simulink model "AC_base_1_VSM_2"  (R2023a)
settings: Solver=ode3  StartTime=0.0  StopTime=8  FixedStep=HWSampleTime  RelTol=1e-3
values from neighbouring files (symbols this model uses):
  ControlSampleTime = 1/8000    (= 0.000125)    [initTPHardware.m]
  HWSampleTime = ControlSampleTime / Oversample    [Sim_TP3_VSM_init.m]    (also in initTPHardware.m = 3.125e-05)
  Ipwm_back = 1.2    [Sim_TP3_VSM_init.m]
  Ipwm_off = 1.2    [Sim_TP3_VSM_init.m]
  Oversample = 1    [Sim_TP3_VSM_init.m]
  scaling_factor = 1/15e4    (= 6.66666666667e-06)    [Sim_TP3_VSM_init.m]
  SM = initStateMachine(EXEC_MODE)    [Sim_TP3_VSM_init.m]
  Ts = ControlSampleTime    [Sim_TP3_VSM_init.m]
  V_DC = 720    [Sim_TP3_VSM_init.m]
undefined symbols (not defined in the file or in its folder): DiscIntNeverNeededParam, LCL, Manage, Param, VSMCTRL
libraries: fl_lib x100, nesl_utility x63, simulink x38, FriedrichLibrary x38, ee_lib x20, simulink_extras x14, TriphaseHardwaremodule x12, spsEdgeDetectorLib x2, StateMachines x2, slpidlib x2, spsPower3phInstantaneousLib x1
(part 3 of 7)

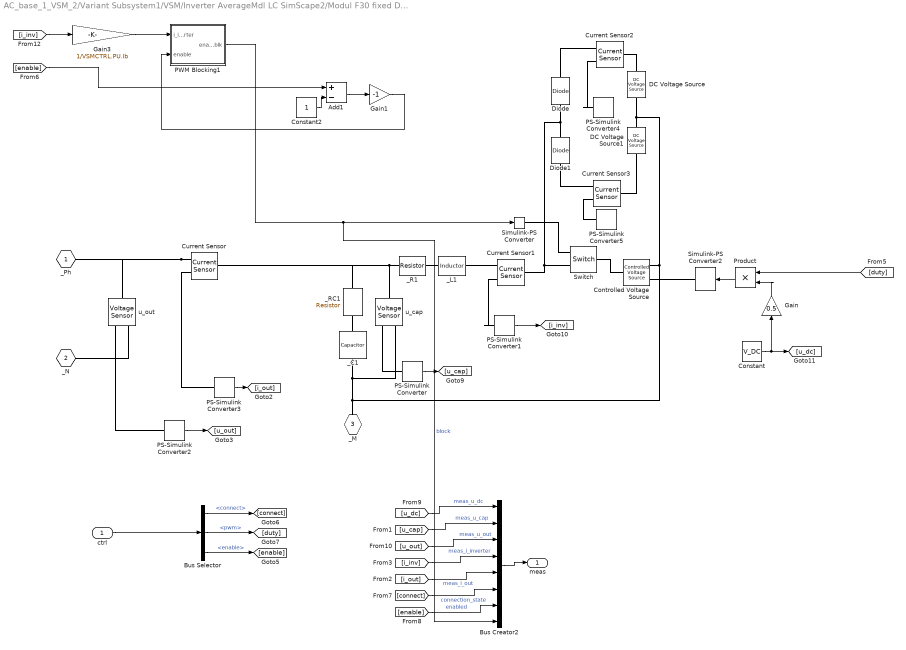
== system AC_base_1_VSM_2/Variant Subsystem1/VSM/Inverter AverageMdl LC SimScape2/Modul F30 fixed DC voltage Average SimScape/simscape_bridgefilter_aca2 ==
  ctrl : Inport
  Add1 : Sum  Inputs=+-
  Bus Creator2 : BusCreator  Inputs=8
  Bus Selector : BusSelector  OutputSignals=connect,pwm,enable
  Constant : Constant  Value=V_DC
  Constant2 : Constant
  Controlled Voltage Source : fl_lib/Electrical/Electrical Sources/Controlled Voltage Source
  Current Sensor{,1..3} (4 alike) : fl_lib/Electrical/Electrical Sensors/Current Sensor
  DC Voltage Source : fl_lib/Electrical/Electrical Sources/DC Voltage Source  v0=V_DC/2 V
  DC Voltage Source1 : fl_lib/Electrical/Electrical Sources/DC Voltage Source  v0=V_DC/2 V
  Diode : fl_lib/Electrical/Electrical Elements/Diode  Vf=0.6 V  Ron=0.001*scaling_factor Ohm  Goff=1e-8 1/Ohm  i_specify=off  i_priority=None  i=0 A  i_nominal_specify=off  i_nominal_unit=A  i_nominal_value=1  v_specify=off  v_priority=None  v=0 V  v_nominal_specify=off  v_nominal_unit=V  v_nominal_value=1
  Diode1 : fl_lib/Electrical/Electrical Elements/Diode  Vf=0.6 V  Ron=0.001*scaling_factor Ohm  Goff=1e-8 1/Ohm  i_specify=off  i_priority=None  i=0 A  i_nominal_specify=off  i_nominal_unit=A  i_nominal_value=1  v_specify=off  v_priority=None  v=0 V  v_nominal_specify=off  v_nominal_unit=V  v_nominal_value=1
  Gain : Gain  Gain=0.5
  Gain1 : Gain  Gain=-1
  Gain3 : Gain  Gain=1/VSMCTRL.PU.Ib
  PS-Simulink Converter{,1..5} (6 alike) : nesl_utility/PS-Simulink Converter  PhysicalDomain=network_engine_domain  SubClassName=ps_output  LeftPortType=input  RightPortType=output  PseudoPeriodic=off  Frequencies=[]  VectorFormat=1-D array  Unit=1  AffineConversion=off
  PWM Blocking1 : Subsystem
  Product : Product
  Simulink-PS Converter : nesl_utility/Simulink-PS Converter  PhysicalDomain=network_engine_domain  SubClassName=ps_input  LeftPortType=input  RightPortType=output  PseudoPeriodic=off  Frequencies=[]  NoiseDistribution=none  NoiseParameters=[]  Unit=1  AffineConversion=off  FilteringAndDerivatives=provide  SimscapeFilterOrder=1  InputFilterTimeConstant=0.001  UdotUserProvided=0
  Simulink-PS Converter2 : nesl_utility/Simulink-PS Converter  PhysicalDomain=network_engine_domain  SubClassName=ps_input  LeftPortType=input  RightPortType=output  PseudoPeriodic=off  Frequencies=[]  NoiseDistribution=none  NoiseParameters=[]  Unit=1  AffineConversion=off  FilteringAndDerivatives=zero  SimscapeFilterOrder=1  InputFilterTimeConstant=0.001  UdotUserProvided=1
  Switch : fl_lib/Electrical/Electrical Elements/Switch  R_closed=0.001*scaling_factor Ohm  G_open=1e-8 1/Ohm  Threshold=0.5  i_specify=off  i_priority=None  i=0 A  i_nominal_specify=off  i_nominal_unit=A  i_nominal_value=1  v_specify=off  v_priority=None  v=0 V  v_nominal_specify=off  v_nominal_unit=V  v_nominal_value=1
  _C1 : fl_lib/Electrical/Electrical Elements/Capacitor  c=C1 F  r=1e-6 Ohm  g=0 1/Ohm  i_specify=off  i_priority=None  i=0 A  i_nominal_specify=off  i_nominal_unit=A  i_nominal_value=1  v_specify=off  v_priority=None  v=0 V  v_nominal_specify=off  v_nominal_unit=V  v_nominal_value=1  vc_specify=off  vc_priority=None  vc=0 V  vc_nominal_specify=off  vc_nominal_unit=V  vc_nominal_value=1
  _L1 : fl_lib/Electrical/Electrical Elements/Inductor  l=L1 H  r=0 Ohm  g=1e-9 1/Ohm  i_specify=off  i_priority=None  i=0 A  i_nominal_specify=off  i_nominal_unit=A  i_nominal_value=1  v_specify=off  v_priority=None  v=0 V  v_nominal_specify=off  v_nominal_unit=V  v_nominal_value=1  i_L_specify=off  i_L_priority=None  i_L=0 A  i_L_nominal_specify=off  i_L_nominal_unit=A  i_L_nominal_value=1
  _R1 : fl_lib/Electrical/Electrical Elements/Resistor  R=R_L1 Ohm  i_specify=off  i_priority=None  i=0 A  i_nominal_specify=off  i_nominal_unit=A  i_nominal_value=1  v_specify=off  v_priority=None  v=0 V  v_nominal_specify=off  v_nominal_unit=V  v_nominal_value=1
  _RC1 : fl_lib/Electrical/Electrical Elements/Resistor  R=R_C1 Ohm  i_specify=off  i_priority=None  i=0 A  i_nominal_specify=off  i_nominal_unit=A  i_nominal_value=1  v_specify=off  v_priority=None  v=0 V  v_nominal_specify=off  v_nominal_unit=V  v_nominal_value=1
  u_cap : fl_lib/Electrical/Electrical Sensors/Voltage Sensor
  u_out : fl_lib/Electrical/Electrical Sensors/Voltage Sensor
  _Ph : PMIOPort  Side=Left
  _N : PMIOPort  Port=2  Side=Left
  _M : PMIOPort  Port=3  Side=Right
  meas : Outport  VectorParamsAs1DForOutWhenUnconnected=off
  wires:
  Gain1/1 -> PWM Blocking1/2(enable)
  [enable] -> Add1/1
  PWM Blocking1/1(enable_blk) -> Simulink-PS Converter/1, Bus Creator2/8  "block"
  [i_inv] -> Gain3/1
  Gain3/1 -> PWM Blocking1/1(i_inverter)
  Add1/1 -> Gain1/1
  Constant2/1 -> Add1/2
  PS-Simulink Converter3/1 -> [i_out]
  Gain/1 -> Product/2
  [duty] -> Product/1
  Constant/1 -> Gain/1, [u_dc]
  Product/1 -> Simulink-PS Converter2/1
  PS-Simulink Converter2/1 -> [u_out]
  PS-Simulink Converter1/1 -> [i_inv]
  PS-Simulink Converter/1 -> [u_cap]
  [u_dc] -> Bus Creator2/1  "meas_u_dc"
  Bus Creator2/1 -> meas/1
  [enable] -> Bus Creator2/7  "enabled"
  Bus Selector/3 -> [enable]  "<enable>"
  [u_cap] -> Bus Creator2/2  "meas_u_cap"
  [u_out] -> Bus Creator2/3  "meas_u_out"
  [i_inv] -> Bus Creator2/4  "meas_i_inverter"
  [i_out] -> Bus Creator2/5  "meas_i_out"
  ctrl/1 -> Bus Selector/1
  [connect] -> Bus Creator2/6  "connection_state"
  Bus Selector/1 -> [connect]  "<connect>"
  Bus Selector/2 -> [duty]  "<pwm>"
  connections:
  Current Sensor2/LConn1 -- DC Voltage Source/LConn1
  PS-Simulink Converter5/LConn1 -- Current Sensor3/RConn1
  Current Sensor2/RConn2 -- Diode/RConn1
  PS-Simulink Converter4/LConn1 -- Current Sensor2/RConn1
  Current Sensor3/RConn2 -- Diode1/LConn1
  Current Sensor3/LConn1 -- DC Voltage Source1/RConn1
  Simulink-PS Converter/RConn1 -- Switch/RConn1
  Controlled Voltage Source/LConn1 -- Switch/LConn1
  Diode/LConn1 -- Switch/RConn2 -- Current Sensor1/LConn1 -- Diode1/RConn1
  _RC1/RConn1 -- _C1/LConn1
  PS-Simulink Converter3/LConn1 -- Current Sensor/RConn1
  PS-Simulink Converter2/LConn1 -- u_out/RConn1
  PS-Simulink Converter1/LConn1 -- Current Sensor1/RConn1
  PS-Simulink Converter/LConn1 -- u_cap/RConn1
  Simulink-PS Converter2/RConn1 -- Controlled Voltage Source/RConn1
  u_out/RConn2 -- _N/RConn1
  Current Sensor/RConn2 -- _Ph/RConn1 -- u_out/LConn1
  DC Voltage Source1/LConn1 -- Controlled Voltage Source/RConn2 -- _C1/RConn1 -- u_cap/RConn2 -- _M/RConn1 -- DC Voltage Source/RConn1
  _R1/LConn1 -- u_cap/LConn1 -- Current Sensor/LConn1 -- _RC1/LConn1
  Current Sensor1/RConn2 -- _L1/RConn1
  _R1/RConn1 -- _L1/LConn1

== system AC_base_1_VSM_2/Variant Subsystem1/VSM/VSM1/VSM/BUS_GENERATION ==
  MANAGE : Inport
  CONTROL : Inport  Port=2
  Bus Creator1 : BusCreator  Inputs=4
  Bus Selector2 : BusSelector  OutputSignals=PWM
  Bus Selector3 : BusSelector  OutputSignals=ENABLED,CONNECT
  Bus Selector4 : BusSelector  OutputSignals=CONNECTED,ENABLED
  Bus Creator6 : BusCreator  Inputs=2  OutDataTypeStr=Bus: FeedbackACBus
  Data Type Conversion{,1..3} (4 alike) : DataTypeConversion  SaturateOnIntegerOverflow=off  RndMeth=Floor
  Signal Specification1 : SignalSpecification
  additional data1 : Constant  Value=0
  ctrl : Outport  VectorParamsAs1DForOutWhenUnconnected=off
  feedback : Outport  Port=2  VectorParamsAs1DForOutWhenUnconnected=off
  wires:
  Bus Selector2/1 -> Signal Specification1/1  "<PWM>"
  Bus Selector4/1 -> Data Type Conversion3/1  "<CONNECTED>"
  Bus Selector4/2 -> Data Type Conversion2/1  "<ENABLED>"
  CONTROL/1 -> Bus Selector2/1
  Data Type Conversion2/1 -> Bus Creator6/2  "enabled"
  Signal Specification1/1 -> Bus Creator1/1  "pwm"
  MANAGE/1 -> Bus Selector3/1, Bus Selector4/1
  Bus Creator1/1 -> ctrl/1
  Bus Creator6/1 -> feedback/1
  Bus Selector3/1 -> Data Type Conversion/1  "<ENABLED>"
  Data Type Conversion/1 -> Bus Creator1/2  "enable"
  Data Type Conversion1/1 -> Bus Creator1/3  "connect"
  additional data1/1 -> Bus Creator1/4  "source_id"
  Bus Selector3/2 -> Data Type Conversion1/1  "<CONNECT>"
  Data Type Conversion3/1 -> Bus Creator6/1  "connected"

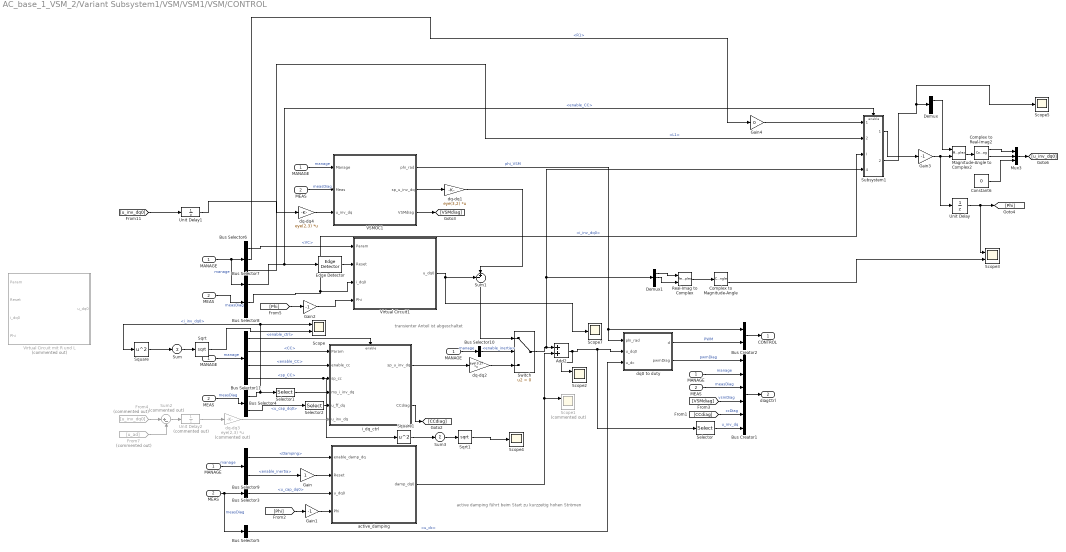
== system AC_base_1_VSM_2/Variant Subsystem1/VSM/VSM1/VSM/CONTROL ==
  note: transienter Anteil ist abgeschaltet
  note: active damping führt beim Start zu kurzzeitig hohen Strömen
  MANAGE : Inport
  MEAS : Inport  Port=2
  "  MANAGE " : InportShadow
  "  MEAS " : InportShadow  Port=2
  "  MEAS  " : InportShadow  Port=2
  " MANAGE" : InportShadow
  " MEAS" : InportShadow  Port=2
  Add2 : Sum
  Bus Creator1 : BusCreator  Inputs=6
  Bus Creator2 : BusCreator  Inputs=2
  Bus Selector10 : BusSelector  OutputSignals=enable_VSM.enable_inertia
  Bus Selector11 : BusSelector  OutputSignals=enable_VSM.enable_ctrl,Param.CC,enable_CC,sp_CC
  Bus Selector3 : BusSelector  OutputSignals=u_cap.u_cap_dq0
  Bus Selector4 : BusSelector  OutputSignals=i_inv.i_inv_dq0,u_cap.u_cap_dq0
  Bus Selector5 : BusSelector  OutputSignals=u_dc
  Bus Selector6 : BusSelector  OutputSignals=Param.VC,Param.VC.R1,Param.VC.L1
  Bus Selector7 : BusSelector  OutputSignals=enable_CC
  Bus Selector8 : BusSelector  OutputSignals=i_inv.i_inv_dq0
  Bus Selector9 : BusSelector  OutputSignals=Param.Damping,enable_VSM.enable_inertia
  Complex to Magnitude-Angle : ComplexToMagnitudeAngle
  Complex to Real-Imag2 : ComplexToRealImag
  Constant6 : Constant  Value=0
  Demux : Demux  Outputs=2
  Demux1 : Demux  Outputs=3
  Edge Detector : spsEdgeDetectorLib/Edge Detector  model=Falling  ic=0  Ts=0
  From4 : From  Commented=on  GotoTag=u_inv_dq0
  From7 : From  Commented=on  GotoTag=u_ad
  Gain : Gain
  Gain1 : Gain  Gain=-1
  Gain2 : Gain  Gain=-1
  Gain3 : Gain  Gain=-1
  Gain4 : Gain  Gain=0
  "MANAGE  " : InportShadow
  "MANAGE   " : InportShadow
  "MANAGE    " : InportShadow
  "MEAS " : InportShadow  Port=2
  Magnitude-Angle to Complex2 : MagnitudeAngleToComplex
  Mux3 : Mux  Inputs=3
  Real-Imag to Complex : RealImagToComplex
  Scope : Scope  NumInputPorts=2
  Scope1 : Scope  Commented=on  NumInputPorts=2
  Scope2 : Scope  NumInputPorts=2
  Scope3 : Scope  NumInputPorts=2
  Scope4 : Scope
  Scope5 : Scope
  Scope7 : Scope  NumInputPorts=3
  Selector : Selector  InputPortWidth=3  IndexOptions=Index vector (dialog)  Indices=[1 2]  OutputSizes=1
  Selector1 : Selector  InputPortWidth=3  IndexOptions=Index vector (dialog)  Indices=[1 2]  OutputSizes=1
  Selector2 : Selector  InputPortWidth=3  IndexOptions=Index vector (dialog)  Indices=[1 2]  OutputSizes=1
  Sqrt : Sqrt
  Sqrt1 : Sqrt
  Square : Math  Operator=square
  Square1 : Math  Operator=square
  Subsystem1 : Subsystem
  Sum : Sum  Inputs=+
  Sum1 : Sum  Inputs=-+|
  Sum2 : Sum  Commented=on  Inputs=|+-
  Sum3 : Sum  Inputs=+
  Switch : Switch  Criteria=u2 > Threshold  SaturateOnIntegerOverflow=off  InputSameDT=off
  Unit Delay : UnitDelay  SampleTime=-1  HasFrameUpgradeWarning=on
  Unit Delay1 : UnitDelay  SampleTime=ControlSampleTime  HasFrameUpgradeWarning=on
  Unit Delay2 : UnitDelay  Commented=on  SampleTime=ControlSampleTime  HasFrameUpgradeWarning=on
  VSMOC1 : Subsystem  mask(VSM mit OC){VSM=Ctrl.VSM}
      mask prompts: VSM "VSM Parameter"
      mask help:
      | VSM(.Ta, .kpf, .kdf, .f0, .ku, .Tu)
      |
      | Parameter nicht auf der Maske:
      | ControlSampleTime
  Virtual Circuit mit R und L : Subsystem  Commented=on  AncestorBlock=ControLibrary/Virtual Circuit
      settings: LibrarySourceBlock=ControLibrary/Virtual Circuit
  Virtual Circuit1 : Subsystem  AncestorBlock=ControLibrary/Virtual Circuit
      settings: LibrarySourceBlock=ControLibrary/Virtual Circuit
  active_damping : Subsystem  mask(Lead Lag){OmLead=Ctrl.VTFF.OmLead, OmLag=Ctrl.VTFF.OmLag}
      mask prompts: OmLead "Omega Lead"; OmLag "Omega Lag"
  dq-dq1 : Gain  Gain=eye(3,2)  Multiplication=Matrix(K*u)
  dq-dq2 : Gain  Gain=eye(3,2)  Multiplication=Matrix(K*u)
  dq-dq3 : Gain  Commented=on  Gain=eye(2,3)  Multiplication=Matrix(K*u)
  dq-dq4 : Gain  Gain=eye(2,3)  Multiplication=Matrix(K*u)
  dq0 to duty : Subsystem
  i_dq_ctrl : Subsystem  mask(PI DQ Stromregler){Kp=Ctrl.CC.kp*0+0.28*2.5/2, Ki=Ctrl.CC.ki*0+28*20/2, L_inv=Ctrl.CC.xff, Kff=Ctrl.CC.Kff}
      mask prompts: Kp "P-Anteil:"; Ki "I-Anteil:"; L_inv "Induktivität [pu]:"; Kff "Vorsteuerung"
      mask help:
      | - in pu Einheiten
      | - 2-phasige DQ Regelung
      | - Entkopplung der d- und q-Achse
      | - Vorsteuerung der Kondensatorspannung
      | - Aktive Dämpfung der LC-Filter Resonanz
      | - Aktive Dämpfung der Zwischenkreis Spannung
  CONTROL : Outport  VectorParamsAs1DForOutWhenUnconnected=off
  diagCtrl : Outport  Port=2  VectorParamsAs1DForOutWhenUnconnected=off
  wires:
  Square1/1 -> Sum3/1
  Sum3/1 -> Sqrt1/1
  Sqrt1/1 -> Scope4/1
  Complex to Magnitude-Angle/2 -> Scope3/2
  Real-Imag to Complex/1 -> Complex to Magnitude-Angle/1
  Demux1/1 -> Real-Imag to Complex/1
  Demux1/2 -> Real-Imag to Complex/2
  Unit Delay/1 -> [Phi], Scope3/1
  Sqrt/1 -> Scope/2
  Sum/1 -> Sqrt/1
  Square/1 -> Sum/1
  Gain4/1 -> Subsystem1/1(<R1>)
  Edge Detector/1 -> Virtual Circuit1/2(Reset)
  Demux/1 -> Magnitude-Angle to Complex2/1
  active_damping/1(damp_dq0) -> Add2/2, Scope1/1
  Complex to Real-Imag2/2 -> Mux3/2
  Complex to Real-Imag2/1 -> Mux3/1
  Switch/1 -> Add2/1, Subsystem1/4(U_i), Demux1/1
  i_dq_ctrl/1(sp_u_inv_dq) -> dq-dq2/1
  Gain3/1 -> Magnitude-Angle to Complex2/2, Unit Delay/1
  dq-dq4/1 -> VSMOC1/3(u_inv_dq)
  Subsystem1/2(U_v) -> Demux/1, Scope5/1
  Subsystem1/1(phi_vsm) -> Gain3/1
  dq-dq1/1 -> Sum1/2
  Mux3/1 -> [u_inv_dq0]
  Constant6/1 -> Mux3/3
  Magnitude-Angle to Complex2/1 -> Complex to Real-Imag2/1
  [u_inv_dq0] -> Unit Delay1/1
  Bus Selector6/3 -> Subsystem1/2(<L1>)  "<L1>"
  Bus Selector6/2 -> Gain4/1  "<R1>"
  Virtual Circuit1/1(" u_dq0") -> Sum1/1, Scope7/2
  Bus Selector7/1 -> Subsystem1/Enable, Edge Detector/1  "<enable_CC>"
  Bus Selector8/1 -> Subsystem1/3(I), Virtual Circuit1/3(i_dq0)  "<i_inv_dq0>"
  Bus Selector11/4 -> i_dq_ctrl/3(sp_cc), Square1/1  "<sp_CC>"
  Selector1/1 -> i_dq_ctrl/4(ms_i_inv_dq)
  Bus Selector4/2 -> Selector2/1  "<u_cap_dq0>"
  Bus Selector11/3 -> i_dq_ctrl/2(enable_cc)  "<enable_CC>"
  Gain2/1 -> Virtual Circuit1/4(Phi)
  [Phi] -> Gain2/1
  From7/1 -> Sum2/2
  From4/1 -> Sum2/1
  Sum2/1 -> Unit Delay2/1
  Gain1/1 -> active_damping/4(Phi)
  Gain/1 -> active_damping/2(Reset)
  Bus Selector9/2 -> Gain/1  "<enable_inertia>"
  Bus Selector3/1 -> active_damping/3(u_dq0)  "<u_cap_dq0>"
  Unit Delay2/1 -> dq-dq3/1
  VSMOC1/1(phi_rad) -> dq0 to duty/1(phi_rad), Bus Creator2/1  "phi_VSM"
  Bus Selector6/1 -> Virtual Circuit1/1(Param)  "<VC>"
  "MANAGE   "/1 -> Bus Selector6/1, Bus Selector7/1  "manage"
  "  MEAS  "/1 -> Bus Selector8/1  "measDiag"
  Selector/1 -> Bus Creator1/6  "u_inv_dq"
  VSMOC1/2(sp_u_inv_dq) -> dq-dq1/1
  Bus Selector5/1 -> dq0 to duty/3(u_dc)  "<u_dc>"
  [CCdiag] -> Bus Creator1/5  "ccDiag"
  "MANAGE  "/1 -> Bus Selector10/1  "manage"
  Bus Selector10/1 -> Switch/2  "<enable_inertia>"
  i_dq_ctrl/2(CCdiag) -> [CCdiag]
  Bus Selector4/1 -> Selector1/1, Scope/1, Square/1  "<i_inv_dq0>"
  "MEAS "/1 -> Bus Selector4/1  "measDiag"
  "MANAGE    "/1 -> Bus Selector11/1  "manage"
  Bus Selector11/1 -> i_dq_ctrl/Enable  "<enable_ctrl>"
  Selector2/1 -> i_dq_ctrl/5(u_ff_dq)
  Bus Selector11/2 -> i_dq_ctrl/1(Param)  "<CC>"
  dq-dq3/1 -> i_dq_ctrl/6(u_inv_dq)
  Add2/1 -> dq0 to duty/2(u_dq0), Selector/1, Scope2/1
  MEAS/1 -> VSMOC1/2(Meas)  "measDiag"
  Bus Creator2/1 -> CONTROL/1
  " MEAS"/1 -> Bus Selector5/1, Bus Selector3/1  "measDiag"
  "  MANAGE "/1 -> Bus Creator1/2  "manage"
  Bus Creator1/1 -> diagCtrl/1
  Bus Selector9/1 -> active_damping/1(enable_damp_dq)  "<Damping>"
  " MANAGE"/1 -> Bus Selector9/1  "manage"
  dq0 to duty/2(pwmDiag) -> Bus Creator1/1  "pwmDiag"
  MANAGE/1 -> VSMOC1/1(Manage)  "manage"
  dq0 to duty/1(d) -> Bus Creator2/2  "PWM"
  VSMOC1/3(VSMdiag) -> [VSMdiag]
  "  MEAS "/1 -> Bus Creator1/3  "measDiag"
  [VSMdiag] -> Bus Creator1/4  "vsmDiag"
  Sum1/1 -> Switch/1
  dq-dq2/1 -> Switch/3
  Unit Delay1/1 -> dq-dq4/1
  [Phi] -> Gain1/1

== system AC_base_1_VSM_2/Variant Subsystem1/VSM/VSM1/VSM/MANAGEMENT ==
  CMD : Inport
  MEAS : Inport  Port=2
  "    MEAS   " : InportShadow  Port=2
  "  CMD  " : InportShadow
  " CMD" : InportShadow
  Add : Sum
  Bus Creator4 : BusCreator  Inputs=8
  Bus Creator5 : BusCreator  Inputs=2
  Bus Selector1 : BusSelector  OutputSignals=Param
  Bus Selector3 : BusSelector  OutputSignals=i_inv.i_inv_ab0,i_inv.i_inv_dq0
  Bus Selector7 : BusSelector  OutputSignals=i_inv.i_inv_dq0,PQ,u_cap.u_cap_ab0,PQ_out,i_out.i_out_ab0
  Bus Selector10 : BusSelector  OutputSignals=Param.CC.i_sp_gain
  Bus Selector11 : BusSelector  OutputSignals=Manage.enable
  Bus Selector12 : BusSelector  OutputSignals=Param.CC.ex_stop_cc,Param.CC.ex_start_cc,Param.CC.watchdog.activate,Param.CC.watchdog.abs_i_set,Param.CC.watchdog.abs_i_reset
  Bus Selector13 : BusSelector  OutputSignals=Manage.connect
  Bus Selector14 : BusSelector  OutputSignals=connection_state
  Compare To Constant1 : simulink/Logic and Bit Operations/Compare To Constant  relop===  const=1  OutDataTypeStr=boolean
  Constant1 : Constant  Value=0
  Logical Operator{1,3,5,8..9} (5 alike) : Logic  AllPortsSameDT=off  OutDataTypeStr=boolean
  Logical Operator4 : Logic  Operator=NOT  AllPortsSameDT=off  OutDataTypeStr=boolean
  Logical Operator6 : Logic  Operator=OR  AllPortsSameDT=off  OutDataTypeStr=boolean
  Logical Operator7 : Logic  Operator=NOT  AllPortsSameDT=off  OutDataTypeStr=boolean
  Logical Operator10 : Logic  Inputs=1  AllPortsSameDT=off  OutDataTypeStr=boolean
  "MEAS " : InportShadow  Port=2
  Selector1 : Selector  InputPortWidth=3  IndexOptions=Index vector (dialog)  Indices=[1 2]  OutputSizes=1
  Selector2 : Selector  InputPortWidth=3  IndexOptions=Index vector (dialog)  Indices=[1 2]  OutputSizes=1
  Signal Specification1 : SignalSpecification
  Signal Specification5 : SignalSpecification
  Signal Specification6 : SignalSpecification
  Step : Step  Time=7+10  After=-1.2  SampleTime=0
  Subsystem1 : Subsystem
      settings: PortSchema="{\"entries\":[{\"content\":{\"sides\":[{\"content\":{\"connectorIds\":[\"In1\",\"In2\",\"In3\",\"In4\"]},\"type\":\"ConnectorPlacement.EquallySpacedRectSide\",\"uuid\":\"aab35d75-627c-4ffd-9951-e3576d7320db\"},{\"content\":{\"connectorIds\":[\"Out1\",\"Out2\"],\"side\":\"RIGHT\"},\"type\":\"ConnectorPlacement.EquallySpacedRectSide\",\"uuid\":\"99390366-615d-4dc0-a4b9-7a01bc996075\"},{\"content\":{\"connectorIds\":[\"In5\",\"In6\"],\"side\":\"TOP\"},\"type\":\"ConnectorPlacement.EquallySpacedRectSide\",\"uuid\":\"cd480ac8-3fd2-414e-8b74-691c5964b8fa\"},{\"content\":{\"connectorIds\":[],\"side\":\"HIDDEN\"},\"type\":\"ConnectorPlacement.EquallySpacedRectSide\",\"uuid\":\"eb094f38-97b3-4aba-ac5e-ab488d071caa\"}]},\"type\":\"ConnectorPlacement.EquallySpacedConnector\",\"uuid\":\"65637395-8c41-4247-973f-480dfd8a7bba\"}],\"packageUris\":[\"http://schema.mathworks.com/mf0/Connector/R2020b\"],\"version\":\"1.0\"}"
  current_watchdog : Subsystem  Commented=on
  sp_VSM : Subsystem
  MANAGE : Outport  VectorParamsAs1DForOutWhenUnconnected=off
  wires:
  Bus Selector7/5 -> Selector2/1  "<i_out_ab0>"
  Selector2/1 -> Subsystem1/6(i_out_ab)
  Subsystem1/2(sp_CC) -> Bus Creator4/6
  Subsystem1/1(CC) -> Logical Operator6/2
  Bus Selector7/4 -> Subsystem1/4(<PQ_out>)  "<PQ_out>"
  Bus Selector7/3 -> Subsystem1/3(<u_cap_ab0>)  "<u_cap_ab0>"
  Bus Selector7/1 -> Subsystem1/2(<i_inv_dq0>)  "<i_inv_dq0>"
  Selector1/1 -> current_watchdog/3(i_ab), current_watchdog/6(i_inv), Subsystem1/1(i_inv_ab)
  Bus Selector7/2 -> current_watchdog/5(PQ)  "<PQ>"
  Constant1/1 -> current_watchdog/2(|i| reset)  "sp_CC"
  Step/1 -> Add/1
  Add/1 -> current_watchdog/1(|i| set)
  Bus Selector12/4 -> Add/2  "<abs_i_set>"
  Bus Selector1/1 -> Bus Creator4/8  "<Param>"
  sp_VSM/1(sp_VSM) -> Bus Creator4/7  "sp_VSM"
  "    MEAS   "/1 -> Bus Selector7/1, sp_VSM/3(MEAS)
  Bus Selector10/1 -> current_watchdog/4(sp_gain)  "<i_sp_gain>"
  Bus Selector11/1 -> Subsystem1/5(enable), Logical Operator10/1  "<enable>"
  Bus Selector12/3 -> Logical Operator5/2  "<activate>"
  Logical Operator5/1 -> current_watchdog/Enable
  Bus Selector12/1 -> Logical Operator4/1  "<ex_stop_cc>"
  Bus Selector12/2 -> Logical Operator6/1  "<ex_start_cc>"
  "  CMD  "/1 -> Bus Selector10/1, sp_VSM/2(CMD), Bus Selector1/1
  Signal Specification1/1 -> Logical Operator3/1, Bus Creator4/2  "CONNECTED"
  Logical Operator10/1 -> Logical Operator3/2
  Signal Specification6/1 -> Bus Creator4/1  "CONNECT"
  Bus Selector13/1 -> Signal Specification6/1  "<connect>"
  CMD/1 -> Bus Selector13/1
  Compare To Constant1/1 -> Signal Specification1/1
  Logical Operator3/1 -> Logical Operator9/1, sp_VSM/1(EnableRateLimit), Signal Specification5/1, Logical Operator8/1, Bus Creator4/3  "ENABLED"
  MEAS/1 -> Bus Selector14/1
  Bus Selector14/1 -> Compare To Constant1/1  "<connection_state>"
  " CMD"/1 -> Bus Selector12/1, Bus Selector11/1
  Bus Selector3/1 -> Selector1/1  "<i_inv_ab0>"
  Logical Operator6/1 -> Logical Operator1/2
  "MEAS "/1 -> Bus Selector3/1
  Bus Creator4/1 -> MANAGE/1
  Logical Operator8/1 -> Bus Creator4/4  "enable_CC"
  Bus Creator5/1 -> Bus Creator4/5  "enable_VSM"
  Signal Specification5/1 -> Bus Creator5/1  "enable_ctrl"
  Logical Operator9/1 -> Bus Creator5/2  "enable_inertia"
  Logical Operator7/1 -> Logical Operator9/2
  Logical Operator1/1 -> Logical Operator7/1, Logical Operator8/2  "enable_cc"
  Logical Operator4/1 -> Logical Operator1/1, Logical Operator5/1

== system AC_base_1_VSM_2/Variant Subsystem1/VSM/VSM1/VSM/Meas ==
  note: VSM Reference Frame
  note: Ucap reference frame
  MEASIN : Inport
  "CONTROL " : Inport  Port=2
  Bus Creator : BusCreator  Inputs=4
  Bus Creator4 : BusCreator  Inputs=10
  Bus Selector : BusSelector  OutputSignals=meas_i_inverter,meas_u_cap,meas_u_out,meas_i_out,meas_vol_dc
  Bus Selector1 : BusSelector  OutputSignals=connection_state,enabled
  Bus Selector2 : BusSelector  OutputSignals=phi_VSM
  Gain{,1..3} (4 alike) : Gain  Gain=eye(3,NrChannels)  Multiplication=Matrix(K*u)
  InstantPowerPhN : FriedrichLibrary/Transformations/InstantPowerPhN  SystemSampleTime=-1  VariantActivationTime=update diagram  Latency=0  AutoFrameSizeCalculation=off
  "InstantPowerPhN " : FriedrichLibrary/Transformations/InstantPowerPhN  SystemSampleTime=-1  VariantActivationTime=update diagram  Latency=0  AutoFrameSizeCalculation=off
  PowerPu : Gain  Gain=2/3
  "PowerPu " : Gain  Gain=2/3
  "SI -> pu" : Subsystem  mask{PU=PU}
      mask prompts: PU "PU System"
      mask DialogControl ParameterGroupVar Prompt: Per Unit
  Signal Specification : SignalSpecification  Dimensions=1
  Signal Specification1 : SignalSpecification  Dimensions=1
  Signal Specification2 : SignalSpecification  Dimensions=3
  Signal Specification3 : SignalSpecification  Dimensions=1
  Symmetrical PLL : FriedrichLibrary/Discrete Stuff/Symmetrical PLL  Kp_PLL=PLL.kp  Ki_PLL=PLL.ki  Kd_PLL=0  Ts=ControlSampleTime
  f2omega : Gain  Gain=2*pi
  meas_i_inv : Subsystem
  meas_i_out : Subsystem
  meas_u_cap : Subsystem
  meas_u_out : Subsystem
  MEAS : Outport  VectorParamsAs1DForOutWhenUnconnected=off
  wires:
  meas_i_out/1(i_out_x) -> Bus Creator4/6  "i_out"
  Gain1/1 -> Symmetrical PLL/1, InstantPowerPhN/1, "InstantPowerPhN "/1, meas_u_cap/1(abc)
  "PowerPu "/1 -> Bus Creator4/9  "PQ_out"
  "InstantPowerPhN "/1 -> "PowerPu "/1
  Bus Selector2/1 -> meas_u_cap/2(phi), meas_u_out/2(phi), meas_i_inv/2(phi)  "<phi_VSM>"
  Bus Selector1/2 -> Bus Creator4/2  "<enabled>"
  Bus Selector1/1 -> Bus Creator4/1  "<connection_state>"
  Bus Creator4/1 -> MEAS/1
  Signal Specification3/1 -> Bus Creator4/10  "u_dc"
  "SI -> pu"/1(MeasOut) -> Bus Selector/1
  f2omega/1 -> Bus Creator/4  "omega"
  Signal Specification2/1 -> Bus Creator/1  "vdq"
  Signal Specification1/1 -> Bus Creator/2  "phi"
  Signal Specification/1 -> Bus Creator/3, f2omega/1  "f"
  "CONTROL "/1 -> Bus Selector2/1
  MEASIN/1 -> "SI -> pu"/1(MeasIn), Bus Selector1/1
  Bus Selector/5 -> Signal Specification3/1  "<meas_vol_dc>"
  Bus Selector/1 -> Gain/1  "<meas_i_inverter>"
  Symmetrical PLL/2 -> meas_i_out/2(phi), Signal Specification1/1  "phi"
  Symmetrical PLL/3 -> Signal Specification/1  "f"
  Symmetrical PLL/1 -> Signal Specification2/1  "vdq"
  Gain/1 -> meas_i_inv/1(abc), InstantPowerPhN/2
  Bus Selector/2 -> Gain1/1  "<meas_u_cap>"
  InstantPowerPhN/1 -> PowerPu/1
  meas_i_inv/1(i_inv_x) -> Bus Creator4/3  "i_inv"
  meas_u_cap/1(u_cap_x) -> Bus Creator4/4  "u_cap"
  Gain2/1 -> "InstantPowerPhN "/2, meas_i_out/1(abc)
  Bus Selector/4 -> Gain2/1  "<meas_i_out>"
  Bus Creator/1 -> Bus Creator4/7  "PLL"
  Bus Selector/3 -> Gain3/1  "<meas_u_out>"
  meas_u_out/1(u_out_x) -> Bus Creator4/5  "u_out"
  Gain3/1 -> meas_u_out/1(abc)
  PowerPu/1 -> Bus Creator4/8  "PQ"

== system AC_base_1_VSM_2/Variant Subsystem1/VSM/VSM1/command_center/Error ACK ==
  Toggle : Constant  OutMin=0  OutMax=1
  Out : Outport  VectorParamsAs1DForOutWhenUnconnected=off
  wires:
  Toggle/1 -> Out/1

== system AC_base_1_VSM_2/Variant Subsystem1/VSM/VSM1/command_center/Shortcut1 ==

== system AC_base_1_VSM_2/Variant Subsystem1/VSM/VSM1/command_center/Subsystem ==
  In1 : Inport
  In2 : Inport  Port=2
  Enable : EnablePort
  Constant : Constant  Value=4
  Display : Display
  TRI - WP : StateMachines/TRI - WP  Time_Pre1=0.3  T_Pre0=0.1  T_Connect=0.3  T_Disconnect=0.1  T_Enable=0.3  T_Disable=0.1  Time_Error=0.1  Ts=SM.TsTimer
  Terminator : Terminator
  Unit Delay : UnitDelay  SampleTime=ControlSampleTime  HasFrameUpgradeWarning=on
  Unit Delay1 : UnitDelay  SampleTime=ControlSampleTime  HasFrameUpgradeWarning=on
  precharge : Outport
  cmd_ac : Outport  Port=2
  wires:
  In2/1 -> Unit Delay1/1
  TRI - WP/2 -> precharge/1  "precharge"
  TRI - WP/1 -> Display/1
  Unit Delay/1 -> TRI - WP/2
  Unit Delay1/1 -> TRI - WP/3
  Constant/1 -> TRI - WP/1
  TRI - WP/4 -> Terminator/1
  In1/1 -> Unit Delay/1
  TRI - WP/3 -> cmd_ac/1

== system AC_base_1_VSM_2/Variant Subsystem1/VSM/VSM1/command_center/cmd_VSM ==
  note: Parameter
  Bus Creator1 : BusCreator  Inputs=4
  Bus Creator2 : BusCreator  Inputs=2
  Current Control : Subsystem
  Damping : Subsystem
  Manage : Subsystem
  Virtual Circuit : Subsystem
  Virtual Synchronous Machine : Subsystem
  cmd_ac : Outport  VectorParamsAs1DForOutWhenUnconnected=off
  wires:
  Bus Creator1/1 -> Bus Creator2/2  "Param"
  Manage/1(Manage) -> Bus Creator2/1  "Manage"
  Virtual Circuit/1(Virtual Circuit) -> Bus Creator1/4  "VC"
  Damping/1(Damping) -> Bus Creator1/3  "Damping"
  Current Control/1(Current Control) -> Bus Creator1/2  "CC"
  Virtual Synchronous Machine/1(Virtual Synchronous Machine) -> Bus Creator1/1  "VSM"
  Bus Creator2/1 -> cmd_ac/1

== system AC_base_1_VSM_2/Variant Subsystem1/VSM/VSM1/diagPlot/dq->abs1 ==
  dq : Inport
  Abs : Abs  SaturateOnIntegerOverflow=off
  Demux : Demux  Outputs=2
  Real-Imag to Complex : RealImagToComplex
  abs : Outport  VectorParamsAs1DForOutWhenUnconnected=off
  wires:
  Demux/1 -> Real-Imag to Complex/1
  Real-Imag to Complex/1 -> Abs/1
  dq/1 -> Demux/1
  Demux/2 -> Real-Imag to Complex/2
  Abs/1 -> abs/1

== system AC_base_1_VSM_2/Variant Subsystem1/VSM/VSM1/diagPlot/dq0->abs ==
  dq0 : Inport
  Abs : Abs  SaturateOnIntegerOverflow=off
  Demux : Demux  Outputs=3
  Real-Imag to Complex : RealImagToComplex
  Terminator : Terminator
  abs : Outport  VectorParamsAs1DForOutWhenUnconnected=off
  wires:
  Abs/1 -> abs/1
  Demux/2 -> Real-Imag to Complex/2
  dq0/1 -> Demux/1
  Real-Imag to Complex/1 -> Abs/1
  Demux/1 -> Real-Imag to Complex/1
  Demux/3 -> Terminator/1

== system AC_base_1_VSM_2/Variant Subsystem1/VSM/VSM1/diagPlot/dq0->abs2 ==
  dq0 : Inport
  Abs : Abs  SaturateOnIntegerOverflow=off
  Demux : Demux  Outputs=3
  Real-Imag to Complex : RealImagToComplex
  Terminator : Terminator
  abs : Outport  VectorParamsAs1DForOutWhenUnconnected=off
  wires:
  Abs/1 -> abs/1
  Demux/2 -> Real-Imag to Complex/2
  dq0/1 -> Demux/1
  Real-Imag to Complex/1 -> Abs/1
  Demux/1 -> Real-Imag to Complex/1
  Demux/3 -> Terminator/1

== system AC_base_1_VSM_2/Variant Subsystem3/VSM/Inverter AverageMdl LC SimScape2/Modul F30 fixed DC voltage Average SimScape/ctrlSelect3 ==
  ctrl : Inport
  Bus Creator1 : BusCreator  Inputs=3
  Bus Creator2 : BusCreator  Inputs=3
  Bus Creator3 : BusCreator  Inputs=3
  Bus Selector : BusSelector  OutputSignals=pwm,connect,enable
  Compare To Constant : simulink/Logic and Bit Operations/Compare To Constant  relop=<  const=0.5  OutDataTypeStr=boolean
  Constant : Constant
  Data Type Conversion : DataTypeConversion  OutDataTypeStr=double  SaturateOnIntegerOverflow=off  RndMeth=Floor
  Data Type Conversion1 : DataTypeConversion  OutDataTypeStr=double  SaturateOnIntegerOverflow=off  RndMeth=Floor
  Rate Transition : RateTransition  Integrity=off  Deterministic=off  OutPortSampleTime=0
  Selector1 : Selector  InputPortWidth=3  IndexOptions=Index vector (dialog)  Indices=[1]  OutputSizes=1
  Selector2 : Selector  InputPortWidth=3  IndexOptions=Index vector (dialog)  Indices=2  OutputSizes=1
  Selector3 : Selector  InputPortWidth=3  IndexOptions=Index vector (dialog)  Indices=3  OutputSizes=1
  Sum of Elements : Sum  Inputs=+
  Sum of Elements1 : Sum  Inputs=+  SampleTime=ControlSampleTime
  ctrl1 : Outport  VectorParamsAs1DForOutWhenUnconnected=off
  ctrl2 : Outport  Port=2  VectorParamsAs1DForOutWhenUnconnected=off
  ctrl3 : Outport  Port=3  VectorParamsAs1DForOutWhenUnconnected=off
  wires:
  Rate Transition/1 -> Selector1/1, Selector3/1, Selector2/1
  Selector1/1 -> Bus Creator1/1  "pwm"
  Bus Creator3/1 -> ctrl2/1
  Selector2/1 -> Bus Creator3/1  "pwm"
  Bus Creator1/1 -> ctrl1/1
  ctrl/1 -> Bus Selector/1
  Bus Creator2/1 -> ctrl3/1
  Selector3/1 -> Bus Creator2/1  "pwm"
  Bus Selector/1 -> Rate Transition/1  "<pwm>"
  Data Type Conversion/1 -> Bus Creator1/3, Bus Creator2/3, Bus Creator3/3  "enable"
  Data Type Conversion1/1 -> Bus Creator2/2, Bus Creator3/2, Bus Creator1/2  "connect"
  Constant/1 -> Sum of Elements/1, Sum of Elements1/1
  Bus Selector/2 -> Data Type Conversion1/1  "<connect>"
  Bus Selector/3 -> Compare To Constant/1  "<enable>"
  Compare To Constant/1 -> Data Type Conversion/1

== system AC_base_1_VSM_2/Variant Subsystem3/VSM/Inverter AverageMdl LC SimScape2/Modul F30 fixed DC voltage Average SimScape/measMerge3 ==
  meas1 : Inport
  meas2 : Inport  Port=2
  meas3 : Inport  Port=3
  measMerge123 : Subsystem
  meas : Outport  VectorParamsAs1DForOutWhenUnconnected=off
  wires:
  meas3/1 -> measMerge123/3(meas3)
  meas2/1 -> measMerge123/2(meas2)
  measMerge123/1(meas) -> meas/1
  meas1/1 -> measMerge123/1(meas1)

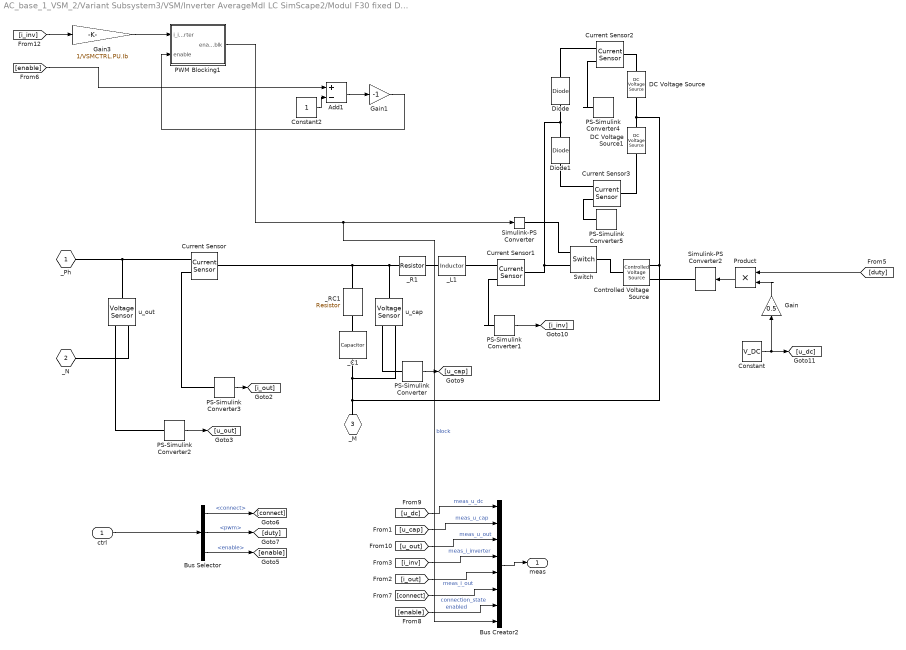
== system AC_base_1_VSM_2/Variant Subsystem3/VSM/Inverter AverageMdl LC SimScape2/Modul F30 fixed DC voltage Average SimScape/simscape_bridgefilter_aca ==
  ctrl : Inport
  Add1 : Sum  Inputs=+-
  Bus Creator2 : BusCreator  Inputs=8
  Bus Selector : BusSelector  OutputSignals=connect,pwm,enable
  Constant : Constant  Value=V_DC
  Constant2 : Constant
  Controlled Voltage Source : fl_lib/Electrical/Electrical Sources/Controlled Voltage Source
  Current Sensor{,1..3} (4 alike) : fl_lib/Electrical/Electrical Sensors/Current Sensor
  DC Voltage Source : fl_lib/Electrical/Electrical Sources/DC Voltage Source  v0=V_DC/2 V
  DC Voltage Source1 : fl_lib/Electrical/Electrical Sources/DC Voltage Source  v0=V_DC/2 V
  Diode : fl_lib/Electrical/Electrical Elements/Diode  Vf=0.6 V  Ron=0.001*scaling_factor Ohm  Goff=1e-8 1/Ohm  i_specify=off  i_priority=None  i=0 A  i_nominal_specify=off  i_nominal_unit=A  i_nominal_value=1  v_specify=off  v_priority=None  v=0 V  v_nominal_specify=off  v_nominal_unit=V  v_nominal_value=1
  Diode1 : fl_lib/Electrical/Electrical Elements/Diode  Vf=0.6 V  Ron=0.001*scaling_factor Ohm  Goff=1e-8 1/Ohm  i_specify=off  i_priority=None  i=0 A  i_nominal_specify=off  i_nominal_unit=A  i_nominal_value=1  v_specify=off  v_priority=None  v=0 V  v_nominal_specify=off  v_nominal_unit=V  v_nominal_value=1
  Gain : Gain  Gain=0.5
  Gain1 : Gain  Gain=-1
  Gain3 : Gain  Gain=1/VSMCTRL.PU.Ib
  PS-Simulink Converter{,1..5} (6 alike) : nesl_utility/PS-Simulink Converter  PhysicalDomain=network_engine_domain  SubClassName=ps_output  LeftPortType=input  RightPortType=output  PseudoPeriodic=off  Frequencies=[]  VectorFormat=1-D array  Unit=1  AffineConversion=off
  PWM Blocking1 : Subsystem
  Product : Product
  Simulink-PS Converter : nesl_utility/Simulink-PS Converter  PhysicalDomain=network_engine_domain  SubClassName=ps_input  LeftPortType=input  RightPortType=output  PseudoPeriodic=off  Frequencies=[]  NoiseDistribution=none  NoiseParameters=[]  Unit=1  AffineConversion=off  FilteringAndDerivatives=provide  SimscapeFilterOrder=1  InputFilterTimeConstant=0.001  UdotUserProvided=0
  Simulink-PS Converter2 : nesl_utility/Simulink-PS Converter  PhysicalDomain=network_engine_domain  SubClassName=ps_input  LeftPortType=input  RightPortType=output  PseudoPeriodic=off  Frequencies=[]  NoiseDistribution=none  NoiseParameters=[]  Unit=1  AffineConversion=off  FilteringAndDerivatives=zero  SimscapeFilterOrder=1  InputFilterTimeConstant=0.001  UdotUserProvided=1
  Switch : fl_lib/Electrical/Electrical Elements/Switch  R_closed=0.001*scaling_factor Ohm  G_open=1e-8 1/Ohm  Threshold=0.5  i_specify=off  i_priority=None  i=0 A  i_nominal_specify=off  i_nominal_unit=A  i_nominal_value=1  v_specify=off  v_priority=None  v=0 V  v_nominal_specify=off  v_nominal_unit=V  v_nominal_value=1
  _C1 : fl_lib/Electrical/Electrical Elements/Capacitor  c=C1 F  r=1e-6 Ohm  g=0 1/Ohm  i_specify=off  i_priority=None  i=0 A  i_nominal_specify=off  i_nominal_unit=A  i_nominal_value=1  v_specify=off  v_priority=None  v=0 V  v_nominal_specify=off  v_nominal_unit=V  v_nominal_value=1  vc_specify=off  vc_priority=None  vc=0 V  vc_nominal_specify=off  vc_nominal_unit=V  vc_nominal_value=1
  _L1 : fl_lib/Electrical/Electrical Elements/Inductor  l=L1 H  r=0 Ohm  g=1e-9 1/Ohm  i_specify=off  i_priority=None  i=0 A  i_nominal_specify=off  i_nominal_unit=A  i_nominal_value=1  v_specify=off  v_priority=None  v=0 V  v_nominal_specify=off  v_nominal_unit=V  v_nominal_value=1  i_L_specify=off  i_L_priority=None  i_L=0 A  i_L_nominal_specify=off  i_L_nominal_unit=A  i_L_nominal_value=1
  _R1 : fl_lib/Electrical/Electrical Elements/Resistor  R=R_L1 Ohm  i_specify=off  i_priority=None  i=0 A  i_nominal_specify=off  i_nominal_unit=A  i_nominal_value=1  v_specify=off  v_priority=None  v=0 V  v_nominal_specify=off  v_nominal_unit=V  v_nominal_value=1
  _RC1 : fl_lib/Electrical/Electrical Elements/Resistor  R=R_C1 Ohm  i_specify=off  i_priority=None  i=0 A  i_nominal_specify=off  i_nominal_unit=A  i_nominal_value=1  v_specify=off  v_priority=None  v=0 V  v_nominal_specify=off  v_nominal_unit=V  v_nominal_value=1
  u_cap : fl_lib/Electrical/Electrical Sensors/Voltage Sensor
  u_out : fl_lib/Electrical/Electrical Sensors/Voltage Sensor
  _Ph : PMIOPort  Side=Left
  _N : PMIOPort  Port=2  Side=Left
  _M : PMIOPort  Port=3  Side=Right
  meas : Outport  VectorParamsAs1DForOutWhenUnconnected=off
  wires:
  Bus Selector/2 -> [duty]  "<pwm>"
  Bus Selector/1 -> [connect]  "<connect>"
  [connect] -> Bus Creator2/6  "connection_state"
  ctrl/1 -> Bus Selector/1
  [i_out] -> Bus Creator2/5  "meas_i_out"
  [i_inv] -> Bus Creator2/4  "meas_i_inverter"
  [u_out] -> Bus Creator2/3  "meas_u_out"
  [u_cap] -> Bus Creator2/2  "meas_u_cap"
  Bus Selector/3 -> [enable]  "<enable>"
  [enable] -> Bus Creator2/7  "enabled"
  Bus Creator2/1 -> meas/1
  [u_dc] -> Bus Creator2/1  "meas_u_dc"
  PS-Simulink Converter/1 -> [u_cap]
  PS-Simulink Converter1/1 -> [i_inv]
  PS-Simulink Converter2/1 -> [u_out]
  Product/1 -> Simulink-PS Converter2/1
  Constant/1 -> [u_dc], Gain/1
  [duty] -> Product/1
  Gain/1 -> Product/2
  PS-Simulink Converter3/1 -> [i_out]
  Constant2/1 -> Add1/2
  Add1/1 -> Gain1/1
  Gain3/1 -> PWM Blocking1/1(i_inverter)
  [i_inv] -> Gain3/1
  PWM Blocking1/1(enable_blk) -> Bus Creator2/8, Simulink-PS Converter/1  "block"
  [enable] -> Add1/1
  Gain1/1 -> PWM Blocking1/2(enable)
  connections:
  _R1/RConn1 -- _L1/LConn1
  Current Sensor1/RConn2 -- _L1/RConn1
  _RC1/LConn1 -- Current Sensor/LConn1 -- u_cap/LConn1 -- _R1/LConn1
  DC Voltage Source/RConn1 -- _M/RConn1 -- u_cap/RConn2 -- _C1/RConn1 -- Controlled Voltage Source/RConn2 -- DC Voltage Source1/LConn1
  u_out/LConn1 -- _Ph/RConn1 -- Current Sensor/RConn2
  u_out/RConn2 -- _N/RConn1
  Simulink-PS Converter2/RConn1 -- Controlled Voltage Source/RConn1
  PS-Simulink Converter/LConn1 -- u_cap/RConn1
  PS-Simulink Converter1/LConn1 -- Current Sensor1/RConn1
  PS-Simulink Converter2/LConn1 -- u_out/RConn1
  PS-Simulink Converter3/LConn1 -- Current Sensor/RConn1
  _RC1/RConn1 -- _C1/LConn1
  Diode1/RConn1 -- Current Sensor1/LConn1 -- Switch/RConn2 -- Diode/LConn1
  Controlled Voltage Source/LConn1 -- Switch/LConn1
  Simulink-PS Converter/RConn1 -- Switch/RConn1
  Current Sensor3/LConn1 -- DC Voltage Source1/RConn1
  Current Sensor3/RConn2 -- Diode1/LConn1
  PS-Simulink Converter4/LConn1 -- Current Sensor2/RConn1
  Current Sensor2/RConn2 -- Diode/RConn1
  PS-Simulink Converter5/LConn1 -- Current Sensor3/RConn1
  Current Sensor2/LConn1 -- DC Voltage Source/LConn1

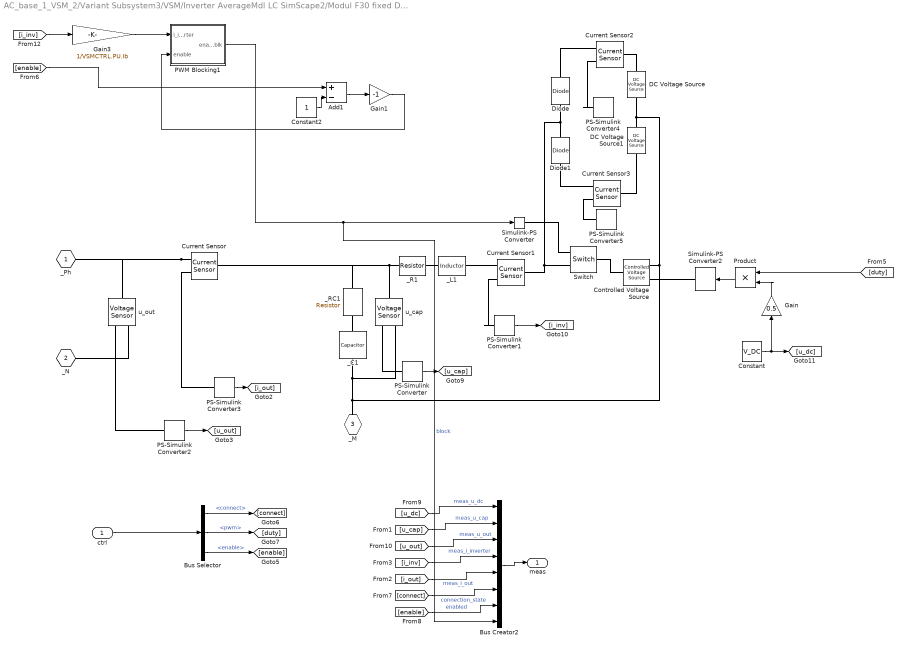
== system AC_base_1_VSM_2/Variant Subsystem3/VSM/Inverter AverageMdl LC SimScape2/Modul F30 fixed DC voltage Average SimScape/simscape_bridgefilter_aca1 ==
  ctrl : Inport
  Add1 : Sum  Inputs=+-
  Bus Creator2 : BusCreator  Inputs=8
  Bus Selector : BusSelector  OutputSignals=connect,pwm,enable
  Constant : Constant  Value=V_DC
  Constant2 : Constant
  Controlled Voltage Source : fl_lib/Electrical/Electrical Sources/Controlled Voltage Source
  Current Sensor{,1..3} (4 alike) : fl_lib/Electrical/Electrical Sensors/Current Sensor
  DC Voltage Source : fl_lib/Electrical/Electrical Sources/DC Voltage Source  v0=V_DC/2 V
  DC Voltage Source1 : fl_lib/Electrical/Electrical Sources/DC Voltage Source  v0=V_DC/2 V
  Diode : fl_lib/Electrical/Electrical Elements/Diode  Vf=0.6 V  Ron=0.001*scaling_factor Ohm  Goff=1e-8 1/Ohm  i_specify=off  i_priority=None  i=0 A  i_nominal_specify=off  i_nominal_unit=A  i_nominal_value=1  v_specify=off  v_priority=None  v=0 V  v_nominal_specify=off  v_nominal_unit=V  v_nominal_value=1
  Diode1 : fl_lib/Electrical/Electrical Elements/Diode  Vf=0.6 V  Ron=0.001*scaling_factor Ohm  Goff=1e-8 1/Ohm  i_specify=off  i_priority=None  i=0 A  i_nominal_specify=off  i_nominal_unit=A  i_nominal_value=1  v_specify=off  v_priority=None  v=0 V  v_nominal_specify=off  v_nominal_unit=V  v_nominal_value=1
  Gain : Gain  Gain=0.5
  Gain1 : Gain  Gain=-1
  Gain3 : Gain  Gain=1/VSMCTRL.PU.Ib
  PS-Simulink Converter{,1..5} (6 alike) : nesl_utility/PS-Simulink Converter  PhysicalDomain=network_engine_domain  SubClassName=ps_output  LeftPortType=input  RightPortType=output  PseudoPeriodic=off  Frequencies=[]  VectorFormat=1-D array  Unit=1  AffineConversion=off
  PWM Blocking1 : Subsystem
  Product : Product
  Simulink-PS Converter : nesl_utility/Simulink-PS Converter  PhysicalDomain=network_engine_domain  SubClassName=ps_input  LeftPortType=input  RightPortType=output  PseudoPeriodic=off  Frequencies=[]  NoiseDistribution=none  NoiseParameters=[]  Unit=1  AffineConversion=off  FilteringAndDerivatives=provide  SimscapeFilterOrder=1  InputFilterTimeConstant=0.001  UdotUserProvided=0
  Simulink-PS Converter2 : nesl_utility/Simulink-PS Converter  PhysicalDomain=network_engine_domain  SubClassName=ps_input  LeftPortType=input  RightPortType=output  PseudoPeriodic=off  Frequencies=[]  NoiseDistribution=none  NoiseParameters=[]  Unit=1  AffineConversion=off  FilteringAndDerivatives=zero  SimscapeFilterOrder=1  InputFilterTimeConstant=0.001  UdotUserProvided=1
  Switch : fl_lib/Electrical/Electrical Elements/Switch  R_closed=0.001*scaling_factor Ohm  G_open=1e-8 1/Ohm  Threshold=0.5  i_specify=off  i_priority=None  i=0 A  i_nominal_specify=off  i_nominal_unit=A  i_nominal_value=1  v_specify=off  v_priority=None  v=0 V  v_nominal_specify=off  v_nominal_unit=V  v_nominal_value=1
  _C1 : fl_lib/Electrical/Electrical Elements/Capacitor  c=C1 F  r=1e-6 Ohm  g=0 1/Ohm  i_specify=off  i_priority=None  i=0 A  i_nominal_specify=off  i_nominal_unit=A  i_nominal_value=1  v_specify=off  v_priority=None  v=0 V  v_nominal_specify=off  v_nominal_unit=V  v_nominal_value=1  vc_specify=off  vc_priority=None  vc=0 V  vc_nominal_specify=off  vc_nominal_unit=V  vc_nominal_value=1
  _L1 : fl_lib/Electrical/Electrical Elements/Inductor  l=L1 H  r=0 Ohm  g=1e-9 1/Ohm  i_specify=off  i_priority=None  i=0 A  i_nominal_specify=off  i_nominal_unit=A  i_nominal_value=1  v_specify=off  v_priority=None  v=0 V  v_nominal_specify=off  v_nominal_unit=V  v_nominal_value=1  i_L_specify=off  i_L_priority=None  i_L=0 A  i_L_nominal_specify=off  i_L_nominal_unit=A  i_L_nominal_value=1
  _R1 : fl_lib/Electrical/Electrical Elements/Resistor  R=R_L1 Ohm  i_specify=off  i_priority=None  i=0 A  i_nominal_specify=off  i_nominal_unit=A  i_nominal_value=1  v_specify=off  v_priority=None  v=0 V  v_nominal_specify=off  v_nominal_unit=V  v_nominal_value=1
  _RC1 : fl_lib/Electrical/Electrical Elements/Resistor  R=R_C1 Ohm  i_specify=off  i_priority=None  i=0 A  i_nominal_specify=off  i_nominal_unit=A  i_nominal_value=1  v_specify=off  v_priority=None  v=0 V  v_nominal_specify=off  v_nominal_unit=V  v_nominal_value=1
  u_cap : fl_lib/Electrical/Electrical Sensors/Voltage Sensor
  u_out : fl_lib/Electrical/Electrical Sensors/Voltage Sensor
  _Ph : PMIOPort  Side=Left
  _N : PMIOPort  Port=2  Side=Left
  _M : PMIOPort  Port=3  Side=Right
  meas : Outport  VectorParamsAs1DForOutWhenUnconnected=off
  wires:
  Gain1/1 -> PWM Blocking1/2(enable)
  [enable] -> Add1/1
  PWM Blocking1/1(enable_blk) -> Simulink-PS Converter/1, Bus Creator2/8  "block"
  [i_inv] -> Gain3/1
  Gain3/1 -> PWM Blocking1/1(i_inverter)
  Add1/1 -> Gain1/1
  Constant2/1 -> Add1/2
  PS-Simulink Converter3/1 -> [i_out]
  Gain/1 -> Product/2
  [duty] -> Product/1
  Constant/1 -> Gain/1, [u_dc]
  Product/1 -> Simulink-PS Converter2/1
  PS-Simulink Converter2/1 -> [u_out]
  PS-Simulink Converter1/1 -> [i_inv]
  PS-Simulink Converter/1 -> [u_cap]
  [u_dc] -> Bus Creator2/1  "meas_u_dc"
  Bus Creator2/1 -> meas/1
  [enable] -> Bus Creator2/7  "enabled"
  Bus Selector/3 -> [enable]  "<enable>"
  [u_cap] -> Bus Creator2/2  "meas_u_cap"
  [u_out] -> Bus Creator2/3  "meas_u_out"
  [i_inv] -> Bus Creator2/4  "meas_i_inverter"
  [i_out] -> Bus Creator2/5  "meas_i_out"
  ctrl/1 -> Bus Selector/1
  [connect] -> Bus Creator2/6  "connection_state"
  Bus Selector/1 -> [connect]  "<connect>"
  Bus Selector/2 -> [duty]  "<pwm>"
  connections:
  Current Sensor2/LConn1 -- DC Voltage Source/LConn1
  PS-Simulink Converter5/LConn1 -- Current Sensor3/RConn1
  Current Sensor2/RConn2 -- Diode/RConn1
  PS-Simulink Converter4/LConn1 -- Current Sensor2/RConn1
  Current Sensor3/RConn2 -- Diode1/LConn1
  Current Sensor3/LConn1 -- DC Voltage Source1/RConn1
  Simulink-PS Converter/RConn1 -- Switch/RConn1
  Controlled Voltage Source/LConn1 -- Switch/LConn1
  Diode/LConn1 -- Switch/RConn2 -- Current Sensor1/LConn1 -- Diode1/RConn1
  _RC1/RConn1 -- _C1/LConn1
  PS-Simulink Converter3/LConn1 -- Current Sensor/RConn1
  PS-Simulink Converter2/LConn1 -- u_out/RConn1
  PS-Simulink Converter1/LConn1 -- Current Sensor1/RConn1
  PS-Simulink Converter/LConn1 -- u_cap/RConn1
  Simulink-PS Converter2/RConn1 -- Controlled Voltage Source/RConn1
  u_out/RConn2 -- _N/RConn1
  Current Sensor/RConn2 -- _Ph/RConn1 -- u_out/LConn1
  DC Voltage Source1/LConn1 -- Controlled Voltage Source/RConn2 -- _C1/RConn1 -- u_cap/RConn2 -- _M/RConn1 -- DC Voltage Source/RConn1
  _R1/LConn1 -- u_cap/LConn1 -- Current Sensor/LConn1 -- _RC1/LConn1
  Current Sensor1/RConn2 -- _L1/RConn1
  _R1/RConn1 -- _L1/LConn1
